simulink model "lcl1"  (R2020a)
settings: Solver=VariableStepAuto  StartTime=0.0  StopTime=.4  RelTol=1e-3
libraries: powerlib x23, powerlib_meascontrol x8, simulink x2, re_lib x1
settings Model: Creator=hp  LastModifiedBy=hp

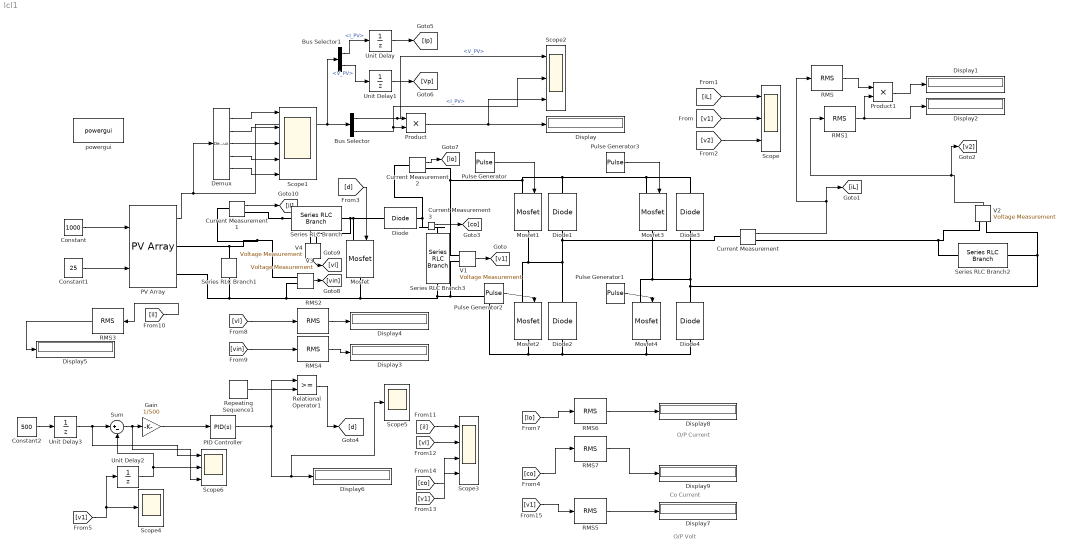
== system lcl1 ==
  note: O/P Volt
  note: Co Current
  note: O/P Current
  Bus Selector : BusSelector  OutputSignals=V_PV,I_PV
  Bus Selector1 : BusSelector  OutputSignals=I_PV,V_PV
  Constant : Constant  Value=1000
  Constant1 : Constant  Value=25
  Constant2 : Constant  Value=500
  Current Measurement{,1..3} (4 alike) : powerlib/Measurements/Current Measurement  PhasorSimulation=off  OutputType=Complex  PSBequivalent=0
  Demux : Demux  Outputs=5  BusSelectionMode=on
  Diode{,1..4} (5 alike) : powerlib/Power Electronics/Diode  Ron=0.001  Lon=0  Vf=0.8  IC=0  UseSnubber=0  Rs=500  Cs=250e-9  Measurements=off
  Display{,1..9} (10 alike) : Display
  Gain : Gain  Gain=1/500
  Mosfet{,1..4} (5 alike) : powerlib/Power Electronics/Mosfet  Ron=0.1  Lon=0  Rd=0.01  Vfd=0  IC=0  Rs=1e5  Cs=inf  Measurements=off
  PID Controller : simulink/Continuous/PID Controller  Controller=PID  Form=Parallel  TimeDomain=Continuous-time  UseExternalTs=off  SampleTime=.02  IntegratorMethod=Forward Euler  FilterMethod=Forward Euler  ControllerParametersSource=internal  P=0  I=-2481.0354  D=0  UseFilter=on  N=100  TunerSelectOption=Frequency Response Based  InitialConditionSource=internal  InitialConditionForIntegrator=0  InitialConditionForFilter=0  DifferentiatorICPrevScaledInput=0  ExternalReset=none  TrackingMode=off  Kt=1  LimitOutput=on  UpperSaturationLimit=0.8307  LowerSaturationLimit=0.3675  LinearizeAsGain=on  AntiWindupMode=none  Kb=1  POutMin=[]  POutMax=[]  IOutMin=[]  IOutMax=[]  DOutMin=[]  DOutMax=[]  NOutMin=[]  NOutMax=[]  SumOutMin=[]  SumOutMax=[]  SaturationOutMin=[]  SaturationOutMax=[]  PParamMin=[]  PParamMax=[]  IParamMin=[]  IParamMax=[]  DParamMin=[]  DParamMax=[]  NParamMin=[]  NParamMax=[]  KbParamMin=[]  KbParamMax=[]  KtParamMin=[]  KtParamMax=[]  KbOutMin=[]  KbOutMax=[]  KtOutMin=[]  KtOutMax=[]  IntegratorOutMin=[]  IntegratorOutMax=[]  FilterOutMin=[]  FilterOutMax=[]  SumI1OutMin=[]  SumI1OutMax=[]  SumI2OutMin=[]  SumI2OutMax=[]  SumI3OutMin=[]  SumI3OutMax=[]  SumI4OutMin=[]  SumI4OutMax=[]  SumDOutMin=[]  SumDOutMax=[]  DifferentiatorOutMin=[]  DifferentiatorOutMax=[]  FilterDiffOutCoefMin=[]  FilterDiffOutCoefMax=[]  ReciprocalOutMin=[]  ReciprocalOutMax=[]  SumDenOutMin=[]  SumDenOutMax=[]  SumNumOutMin=[]  SumNumOutMax=[]  DivideOutMin=[]  DivideOutMax=[]  UdiffTsProdOutMin=[]  UdiffTsProdOutMax=[]  NTsProdOutMin=[]  NTsProdOutMax=[]  UintegralTsProdOutMin=[]  UintegralTsProdOutMax=[]  UngainTsProdOutMin=[]  UngainTsProdOutMax=[]  IntegratorContinuousStateAttributes=''  IntegratorStateMustResolveToSignalObject=off  IntegratorRTWStateStorageClass=Auto  FilterContinuousStateAttributes=''  FilterStateMustResolveToSignalObject=off  FilterRTWStateStorageClass=Auto  ParallelPVariant=InternalParameters  IdealPVariant=Disabled  IVariant=InternalParameters  DVariant=InternalParameters  IntegratorVariant=Continuous  SatVariant=Enabled  AWVariant=Passthrough  PCopyVariant=Disabled  TRVariant=Disabled  FdbkBlocksVariant=Forward  IdealPFdbkVariant=Disabled  SatFdbkVariant=Disabled  DerivativeFilterVariant=ContFilter  NVariant=InternalParameters  NCopyVariant=Disabled  FilterICVariant=InternalICsFilter  IntegratorICVariant=InternalICs  ExternalResetVariant=Disabled  TRSumVariant=Passthrough  SumFdbkVariant=Disabled  SumVariant=Sum_PID  TsampFilterVariant=InternalTs  TsampNgainVariant=Passthrough  TsampIntegralVariant=Passthrough
  PV Array : re_lib/Solar/PV Array  Npar=4  Nser=4  PlotType=array @ 25 deg.C & specified irradiances  S_vec="[ 1000  500  100 50 ]"  Temp_C_vec="[ 45 25  ]"  ModuleName=Centrosolar America BP7-315BW  PlotWhenSelected=off  Pm=315.0042  Ncell=72  Voc=45.45  Isc=8.97  Vm=37.59  Im=8.38  beta_Voc_pc=-0.349  alpha_Isc_pc=0.037001  beta_Voc=-0.15862  alpha_Isc=0.003319  IL=8.9803  I0=1.9823e-10  nI=1.0022  Rsh=237.0635  Rs=0.27147  RobustModel=off  RobustCellTemperature=25  BAL=on  Tc=1e-6  Tfilter=5e-5
  Product : Product
  Product1 : Product
  Pulse Generator : DiscretePulseGenerator  PulseType=Time based  Period=1/(50)  PulseWidth=50  PhaseDelay=0/(360*50)
  Pulse Generator1 : DiscretePulseGenerator  PulseType=Time based  Period=1/(50)  PulseWidth=50  PhaseDelay=0/(360*50)
  Pulse Generator2 : DiscretePulseGenerator  PulseType=Time based  Period=1/(50)  PulseWidth=50  PhaseDelay=180/(360*50)
  Pulse Generator3 : DiscretePulseGenerator  PulseType=Time based  Period=1/(50)  PulseWidth=50  PhaseDelay=180/(360*50)
  RMS{,1..7} (8 alike) : powerlib_meascontrol/Measurements/RMS  TrueRMS=on  Freq=60  RMSInit=120  Ts=0
  Relational Operator1 : RelationalOperator  OutDataTypeStr=boolean  RndMeth=Simplest
  Repeating Sequence1 : simulink/Sources/Repeating Sequence  rep_seq_t=[0 1/(50e3)]  rep_seq_y=[0 1]
  Scope : Scope  NumInputPorts=3
  Scope1 : Scope  NumInputPorts=5
  Scope2 : Scope  NumInputPorts=3
  Scope3 : Scope  NumInputPorts=4
  Scope4 : Scope
  Scope5 : Scope
  Scope6 : Scope  NumInputPorts=3
  Series RLC Branch : powerlib/Elements/Series RLC Branch  LConnTagsString=__new0  RConnTagsString=__new0  BranchType=L  Resistance=1/1000  Inductance=0.0018  SetiL0=off  InitialCurrent=0  Capacitance=1e-6  Setx0=off  InitialVoltage=0  Measurements=None
  Series RLC Branch1 : powerlib/Elements/Series RLC Branch  LConnTagsString=__new0  RConnTagsString=__new0  BranchType=C  Resistance=1/1000  Inductance=1e-3  SetiL0=off  InitialCurrent=0  Capacitance=1.3702e-04  Setx0=on  InitialVoltage=0  Measurements=None
  Series RLC Branch2 : powerlib/Elements/Series RLC Branch  LConnTagsString=__new0  RConnTagsString=__new0  BranchType=R  Resistance=11.22  Inductance=1e-3  SetiL0=off  InitialCurrent=0  Capacitance=1e-6  Setx0=off  InitialVoltage=0  Measurements=None
  Series RLC Branch3 : powerlib/Elements/Series RLC Branch  LConnTagsString=__new0  RConnTagsString=__new0  BranchType=C  Resistance=1/1000  Inductance=1e-3  SetiL0=off  InitialCurrent=0  Capacitance=1.0618e-05  Setx0=on  InitialVoltage=0  Measurements=None
  Sum : Sum  Inputs=|+-
  Unit Delay{,1..3} (4 alike) : UnitDelay  SampleTime=1e-4  HasFrameUpgradeWarning=on
  V{1..4} (4 alike) : powerlib/Measurements/Voltage Measurement  PhasorSimulation=off  OutputType=Complex  PSBequivalent=0
  powergui : powerlib/powergui  Priority=1  SimulationMode=Discrete  SampleTime=50e-8  frequency=60  Iterations=50  frequencyindice=0  Pbase=100e6  ErrMax=1e-4  UnitsV=kV  UnitsW=MW  buscounter=0  FunctionMessages=off  echomessages=off  EnableUseOfTLC=off  CurrentSourceSwitches=off  DisableSnubberDevices=off  DisableRonSwitches=off  DisableVfSwitches=off  DisplayEquations=off  AutomaticDiscreteSolvers=off  SolverType=Tustin/Backward Euler (TBE)  Interpol=off  ExternalGateDelay=off  methode=off  Ts=100  x0status=blocks  SPID=on  SwTol=0  HookPort=off  NonlinearTolerance=1e-4  nMaxIteration=100  ContinueOnMaxIteration=off  RestoreLinks=warning  ResistiveCurrentMeasurement=off  Frange=[0:2:500]  Ylog=off  Xlog=on  ShowGrid=off  save=off  variable=ZData  structure=0  ZoomFFT=off  StartTime=0.0  cycles=1  DisplayStyle=1  fundamental=60  FreqAxis=off  MaxFrequency=1000  frequencyindicesteady=1  RmsSteady=1  display=off
  wires:
  [iL] -> Scope/1
  [v2] -> Scope/3
  Constant1/1 -> PV Array/2
  Demux/2 -> Scope1/2
  Bus Selector/2 -> Scope2/2, Product/2  "<I_PV>"
  Bus Selector/1 -> Scope2/1, Product/1  "<V_PV>"
  Pulse Generator3/1 -> Mosfet3/1
  Pulse Generator2/1 -> Mosfet2/1
  Demux/5 -> Scope1/5
  V1/1 -> [v1]
  Pulse Generator1/1 -> Mosfet4/1
  V2/1 -> [v2], RMS1/1
  Constant/1 -> PV Array/1
  Demux/3 -> Scope1/3
  Demux/1 -> Scope1/1
  Product/1 -> Scope2/3, Display/1
  Pulse Generator/1 -> Mosfet1/1
  Demux/4 -> Scope1/4
  [v1] -> Scope/2
  Bus Selector1/2 -> Unit Delay1/1  "<V_PV>"
  Bus Selector1/1 -> Unit Delay/1  "<I_PV>"
  PV Array/1 -> Demux/1, Bus Selector1/1, Bus Selector/1
  Unit Delay/1 -> [Ip]
  Unit Delay1/1 -> [Vp]
  Product1/1 -> Display1/1
  Current Measurement/1 -> RMS/1, [iL]
  RMS1/1 -> Display2/1, Product1/2
  RMS/1 -> Product1/1
  RMS2/1 -> Display4/1
  RMS3/1 -> Display5/1
  [d] -> Mosfet/1
  RMS4/1 -> Display3/1
  RMS5/1 -> Display7/1
  RMS6/1 -> Display8/1
  RMS7/1 -> Display9/1
  Current Measurement3/1 -> [co]
  Current Measurement2/1 -> [lo]
  V3/1 -> [vin]
  V4/1 -> [vl]
  [vl] -> RMS2/1
  [vin] -> RMS4/1
  Current Measurement1/1 -> [il]
  [il] -> RMS3/1
  [lo] -> RMS6/1
  [co] -> RMS7/1
  [il] -> Scope3/1
  [vl] -> Scope3/2
  [v1] -> Scope3/4
  [co] -> Scope3/3
  [v1] -> RMS5/1
  Sum/1 -> Scope6/3, Gain/1
  [v1] -> Unit Delay2/1, Scope4/1
  PID Controller/1 -> Relational Operator1/1, Scope5/1, Display6/1
  Gain/1 -> PID Controller/1
  Unit Delay2/1 -> Sum/2, Scope6/2
  Repeating Sequence1/1 -> Relational Operator1/2
  Relational Operator1/1 -> [d]
  Constant2/1 -> Unit Delay3/1
  Unit Delay3/1 -> Scope6/1, Sum/1
  connections:
  Series RLC Branch/LConn1 -- Current Measurement1/RConn1 -- V4/LConn1
  Mosfet/LConn1 -- Diode/LConn1 -- V4/LConn2 -- Series RLC Branch/RConn1
  Diode2/RConn1 -- Current Measurement/LConn1 -- Diode1/LConn1 -- Mosfet2/LConn1 -- Mosfet1/RConn1
  Series RLC Branch2/LConn1 -- Current Measurement/RConn1 -- V2/LConn1
  Diode3/LConn1 -- V2/LConn2 -- Series RLC Branch2/RConn1 -- Diode4/RConn1 -- Mosfet3/RConn1 -- Mosfet4/LConn1
  Current Measurement2/LConn1 -- Current Measurement3/LConn1 -- Diode/RConn1
  Mosfet2/RConn1 -- V1/LConn2 -- Mosfet/RConn1 -- Series RLC Branch1/RConn1 -- PV Array/RConn2 -- V3/LConn2 -- Series RLC Branch3/RConn1 -- Diode2/LConn1 -- Diode4/LConn1 -- Mosfet4/RConn1
  V1/LConn1 -- Current Measurement2/RConn1 -- Mosfet1/LConn1 -- Mosfet3/LConn1 -- Diode3/RConn1 -- Diode1/RConn1
  Current Measurement3/RConn1 -- Series RLC Branch3/LConn1
  Current Measurement1/LConn1 -- V3/LConn1 -- Series RLC Branch1/LConn1 -- PV Array/RConn1
